simulink model "DC_Simscape_test_no_graphs"  (R2016a)
settings: Solver=ode23t  StartTime=0.0  StopTime=5790*3  MaxStep=0.1  RelTol=1e-3
libraries: nesl_utility x36, fl_lib x33, elec_lib x8, LiBatteryElements_lib x4
settings Model: Creator=Bruno  LastModifiedBy=sara
settings SolverCC: MaxConsecutiveZCs=10000

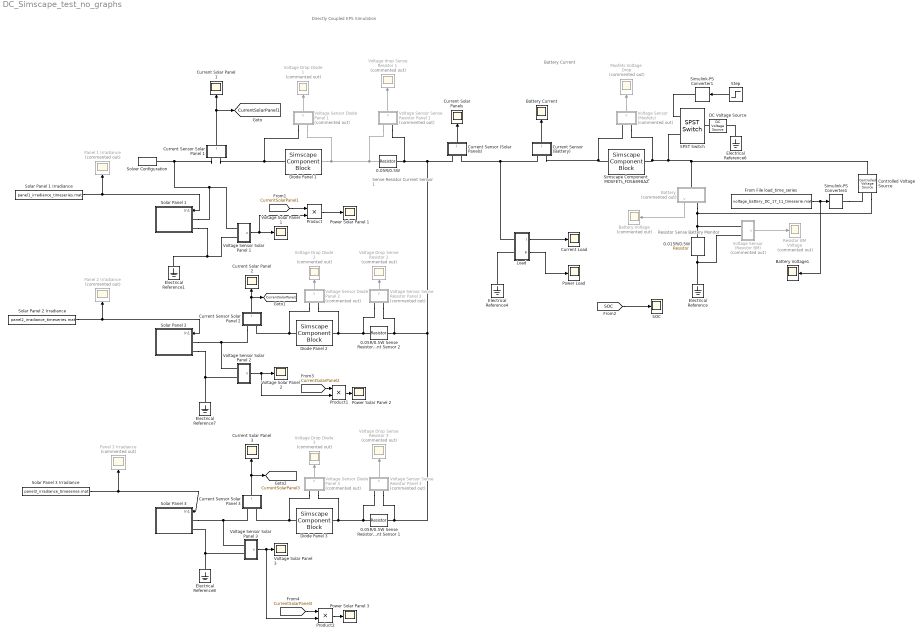
== system DC_Simscape_test_no_graphs ==
  note: Battery Current
  note: Resistor Sense
      | Battery Monitor
  note: Sense Resistor
      | Current Sensor 1
  note: Directly Coupled EPS Simulation
  " Battery" : Subsystem  Commented=on
      settings: CopyFcn=set_param(gcb,'LinkStatus','none')
  " Load" : Subsystem
      settings: CopyFcn=set_param(gcb,'LinkStatus','none')
  " 0.015R/0.5W" : elec_lib/Passive Devices/Resistor  R=0.015 Ohm  R_tol=0.01  enable_R_tol=0  tol_distribution=1  nSigma=4  enable_operating_limits=0  operating_limit_action=2  max_working_voltage=100 V  power_rating=1 W  enable_faults=0  fault_action=1  R_faulted=Inf Ohm  enable_temporal_fault=0  t_fault=1 s  enable_behavioral_fault=0  max_permissible_current=1 A  t_fail_on_current=1 s  noise_mode=0  sample_time=0.001 s  repeatability=1  auto_seed=1471942077  user_seed=0  Tdevice=25 degC  alpha=0.00393 1/K  Tmeas=25 degC  thermal_mass=100 J/K  initial_temperature=25 degC  power_derating_T1=70 degC  power_derating_T2=155 degC  operating_temperature_range_vec=[ -50 150 ] degC
  " 0.05R/0.5W" : elec_lib/Passive Devices/Resistor  R=0.05 Ohm  R_tol=0.01  enable_R_tol=0  tol_distribution=1  nSigma=4  enable_operating_limits=0  operating_limit_action=2  max_working_voltage=100 V  power_rating=1 W  enable_faults=0  fault_action=1  R_faulted=Inf Ohm  enable_temporal_fault=0  t_fault=1 s  enable_behavioral_fault=0  max_permissible_current=1 A  t_fail_on_current=1 s  noise_mode=0  sample_time=0.001 s  repeatability=1  auto_seed=1613585455  user_seed=0  Tdevice=25 degC  alpha=0.00393 1/K  Tmeas=25 degC  thermal_mass=100 J/K  initial_temperature=25 degC  power_derating_T1=70 degC  power_derating_T2=155 degC  operating_temperature_range_vec=[ -50 150 ] degC
  " 0.05R/0.5W Sense Resistor Current Sensor 1" : elec_lib/Passive Devices/Resistor  R=0.05 Ohm  R_tol=0.01  enable_R_tol=0  tol_distribution=1  nSigma=4  enable_operating_limits=0  operating_limit_action=2  max_working_voltage=100 V  power_rating=1 W  enable_faults=0  fault_action=1  R_faulted=Inf Ohm  enable_temporal_fault=0  t_fault=1 s  enable_behavioral_fault=0  max_permissible_current=1 A  t_fail_on_current=1 s  noise_mode=0  sample_time=0.001 s  repeatability=1  auto_seed=4049024516  user_seed=0  Tdevice=25 degC  alpha=0.00393 1/K  Tmeas=25 degC  thermal_mass=100 J/K  initial_temperature=25 degC  power_derating_T1=70 degC  power_derating_T2=155 degC  operating_temperature_range_vec=[ -50 150 ] degC
  " 0.05R/0.5W Sense Resistor Current Sensor 2" : elec_lib/Passive Devices/Resistor  R=0.05 Ohm  R_tol=0.01  enable_R_tol=0  tol_distribution=1  nSigma=4  enable_operating_limits=0  operating_limit_action=2  max_working_voltage=100 V  power_rating=1 W  enable_faults=0  fault_action=1  R_faulted=Inf Ohm  enable_temporal_fault=0  t_fault=1 s  enable_behavioral_fault=0  max_permissible_current=1 A  t_fail_on_current=1 s  noise_mode=0  sample_time=0.001 s  repeatability=1  auto_seed=2353087603  user_seed=0  Tdevice=25 degC  alpha=0.00393 1/K  Tmeas=25 degC  thermal_mass=100 J/K  initial_temperature=25 degC  power_derating_T1=70 degC  power_derating_T2=155 degC  operating_temperature_range_vec=[ -50 150 ] degC
  " Current Solar Panel 1" : Scope
  " Current Solar Panel 2" : Scope
  " Current Solar Panel 3" : Scope
  " Solar Panel 1 Irradiance" : FromFile  FileName=panel1_irradiance_timeseries.mat
  Battery Current : Scope
  Battery Voltage : Scope  Commented=on
  Battery Voltage1 : Scope
  Controlled Voltage Source : fl_lib/Electrical/Electrical Sources/Controlled Voltage Source
  Current Sensor (Battery) : Subsystem
      settings: CopyFcn=set_param(gcb,'LinkStatus','none')
  Current Sensor (Solar Panels) : Subsystem
      settings: CopyFcn=set_param(gcb,'LinkStatus','none')
  Current Sensor Solar Panel 1 : Subsystem
      settings: CopyFcn=set_param(gcb,'LinkStatus','none')
  Current Sensor Solar Panel 2 : Subsystem
      settings: CopyFcn=set_param(gcb,'LinkStatus','none')
  Current Sensor Solar Panel 3 : Subsystem
      settings: CopyFcn=set_param(gcb,'LinkStatus','none')
  Current Solar Panels : Scope
  Current Load : Scope
  DC Voltage Source : fl_lib/Electrical/Electrical Sources/DC Voltage Source  v0=4 V
  Diode Panel 1 : SimscapeComponentBlock  SourceFile=diode_EPS  ComponentPath=diode_EPS  ComponentVariants=diode_EPS  ComponentVariantNames=diode_EPS  ClassName=diode_EPS  SchemaVersion=1  Vt=1.38e-23 * 298 / 1.60e-19 V  R=0.0084 Ohm  n=1.00404  Is=1.3032e-6 A  i_specify=off  i_priority=None  i=1 A  v_specify=off  v_priority=None  v=0 V
      settings: CopyFcn=simscape.engine.sli.internal.componentblockcallback(gcbh,'COPY')  PreCopyFcn=simscape.engine.sli.internal.componentblockcallback(gcbh,'PRECOPY')  PreDeleteFcn=simscape.engine.sli.internal.componentblockcallback(gcbh,'PREDELETE')
      mask Type: Code produced by Embedded Systems Group - UFSC
      mask Display:
      | disp('Simscape\n\n\n')
      | disp('\n\n\ndiode_EPS');
      | color('red');
      | port_label('RConn', 1,'-');
      | port_label('LConn', 1,'+');
  Diode Panel 2 : SimscapeComponentBlock  SourceFile=diode_EPS  ComponentPath=diode_EPS  ComponentVariants=diode_EPS  ComponentVariantNames=diode_EPS  ClassName=diode_EPS  SchemaVersion=1  Vt=1.38e-23 * 298 / 1.60e-19 V  R=0.0084 Ohm  n=1.00404  Is=1.3032e-6 A  i_specify=off  i_priority=None  i=1 A  v_specify=off  v_priority=None  v=0 V
      settings: CopyFcn=simscape.engine.sli.internal.componentblockcallback(gcbh,'COPY')  PreCopyFcn=simscape.engine.sli.internal.componentblockcallback(gcbh,'PRECOPY')  PreDeleteFcn=simscape.engine.sli.internal.componentblockcallback(gcbh,'PREDELETE')
      mask Type: Code produced by Embedded Systems Group - UFSC
      mask Display:
      | disp('Simscape\n\n\n')
      | disp('\n\n\ndiode_EPS');
      | color('red');
      | port_label('RConn', 1,'-');
      | port_label('LConn', 1,'+');
  Diode Panel 3 : SimscapeComponentBlock  SourceFile=diode_EPS  ComponentPath=diode_EPS  ComponentVariants=diode_EPS  ComponentVariantNames=diode_EPS  ClassName=diode_EPS  SchemaVersion=1  Vt=1.38e-23 * 298 / 1.60e-19 V  R=0.0084 Ohm  n=1.00404  Is=1.3032e-6 A  i_specify=off  i_priority=None  i=1 A  v_specify=off  v_priority=None  v=0 V
      settings: CopyFcn=simscape.engine.sli.internal.componentblockcallback(gcbh,'COPY')  PreCopyFcn=simscape.engine.sli.internal.componentblockcallback(gcbh,'PRECOPY')  PreDeleteFcn=simscape.engine.sli.internal.componentblockcallback(gcbh,'PREDELETE')
      mask Type: Code produced by Embedded Systems Group - UFSC
      mask Display:
      | disp('Simscape\n\n\n')
      | disp('\n\n\ndiode_EPS');
      | color('red');
      | port_label('RConn', 1,'-');
      | port_label('LConn', 1,'+');
  Electrical Reference{,1,4,6..8} (6 alike) : fl_lib/Electrical/Electrical Elements/Electrical Reference
  From File load_time_series : FromFile  FileName=voltage_battery_DC_17_11_timeserie.mat  SampleTime=1
  Mosfets Voltage Drop : Scope  Commented=on
  Panel 1 Irradiance : Scope  Commented=on
  Panel 2 Irradiance : Scope  Commented=on
  Panel 3 Irradiance : Scope  Commented=on
  Power Solar Panel 1 : Scope
  Power Solar Panel 2 : Scope
  Power Solar Panel 3 : Scope
  Power Load : Scope
  Product : Product
  Product1 : Product
  Product2 : Product
  Resistor BM Voltage : Scope  Commented=on
  SOC : Scope
  SPST Switch : elec_lib/Passive Devices/Switches/SPST Switch  R_closed=0.01 Ohm  G_open=1e-6 S  Threshold=0 V  Width=0 V  model_dynamics=0  t_on=0.001 s  t_off=0.001 s  initial_vT=0 V
  Simscape Component_MOSFETs_FDS6898AZ : SimscapeComponentBlock  SourceFile=MOSFETs_EPS  ComponentPath=MOSFETs_EPS  ComponentVariants=MOSFETs_EPS  ComponentVariantNames=MOSFETs_EPS  ClassName=MOSFETs_EPS  SchemaVersion=1  Vt=1.38e-23 * 298 / 1.60e-19 V  Rsd=0.27 Ohm  Rs=0.008235 Ohm  n=1.89492  Is=1.26064e-7 A  i_specify=on  i_priority=None  i=1 A  v_specify=on  v_priority=None  v=4 V  Vr_DC_specify=on  Vr_DC_priority=None  Vr_DC=1 V  Vr_CC_specify=on  Vr_CC_priority=None  Vr_CC=1 V
      settings: CopyFcn=simscape.engine.sli.internal.componentblockcallback(gcbh,'COPY')  PreCopyFcn=simscape.engine.sli.internal.componentblockcallback(gcbh,'PRECOPY')  PreDeleteFcn=simscape.engine.sli.internal.componentblockcallback(gcbh,'PREDELETE')
      mask Type: Code produced by Embedded Systems Group - UFSC
      mask Display:
      | disp('Simscape\n\n\n')
      | disp('\n\n\nMOSFETs_EPS');
      | color('red');
      | port_label('RConn', 1,'-');
      | port_label('LConn', 1,'+');
  Simulink-PS Converter1 : nesl_utility/Simulink-PS Converter  PhysicalDomain=network_engine_domain  SubClassName=ps_input  LeftPortType=input  RightPortType=output  PseudoPeriodic=off  Frequencies=[]  NoiseDistribution=none  NoiseParameters=[]  Unit=1  AffineConversion=off  InputFiltering=off  SimscapeFilterOrder=1  InputFilterTimeConstant=0.001  UdotUserProvided=1
  Simulink-PS Converter4 : nesl_utility/Simulink-PS Converter  PhysicalDomain=network_engine_domain  SubClassName=ps_input  LeftPortType=input  RightPortType=output  PseudoPeriodic=off  Frequencies=[]  NoiseDistribution=none  NoiseParameters=[]  Unit=1  AffineConversion=off  InputFiltering=off  SimscapeFilterOrder=1  InputFilterTimeConstant=0.001  UdotUserProvided=1
  Solar Panel 1 : Subsystem
      settings: CopyFcn=set_param(gcb,'LinkStatus','none')
  Solar Panel 2 : Subsystem
      settings: CopyFcn=set_param(gcb,'LinkStatus','none')
  Solar Panel 2 Irradiance : FromFile  FileName=panel2_irradiance_timeseries.mat
  Solar Panel 3 : Subsystem
      settings: CopyFcn=set_param(gcb,'LinkStatus','none')
  Solar Panel 3 Irradiance : FromFile  FileName=panel3_irradiance_timeseries.mat
  Solver Configuration : nesl_utility/Solver Configuration  PhysicalDomain=network_engine_domain  SubClassName=solver  LeftPortType=input  RightPortType=generic  Accelerate=off  Tones=[]  Harmonics=[]  SimulateNoise=off  Profile=off  UseLocalSampling=off  EnableSwitchedLinearOptims=on  FrequencyDomain=off  UseCCode=off  RelTol=0.001  AbsTol=1e-06  MinStep=1e-09  ToWorkspace=off  RevertToSquareIcSolve=off  NumHomotopyIterations=100  PhasorMode=off  PhasorModeNumHarmonics=1  OverrideAbsTol=off  DoDC=off  ResidualTolerance=1e-3  UseLocalSolver=off  LocalSolverChoice=NE_BACKWARD_EULER_ADVANCER  LocalSolverSampleTime=.001  DoFixedCost=off  MaxNonlinIter=3  MaxModeIter=2  LinearAlgebra=Sparse  DelaysMemoryBudget=1024  AutomaticFiltering=on  FilteringTimeConstant=0.001
  Step : Step  Before=1  After=0  SampleTime=0
  Voltage Sensor (Mosfets) : Subsystem  Commented=on
      settings: CopyFcn=set_param(gcb,'LinkStatus','none')
  Voltage Sensor (Resistor BM) : Subsystem  Commented=on
      settings: CopyFcn=set_param(gcb,'LinkStatus','none')
  Voltage Solar Panel 1 : Scope
  Voltage Solar Panel 2 : Scope
  Voltage Solar Panel 3 : Scope
  "Voltage Drop Diode 1 " : Scope  Commented=on
  Voltage Drop Diode 2 : Scope  Commented=on
  Voltage Drop Diode 3 : Scope  Commented=on
  Voltage Drop Sense Resistor 2 : Scope  Commented=on
  Voltage Drop Sense Resistor 3 : Scope  Commented=on
  Voltage Sensor Diode Panel 1 : Subsystem  Commented=on
      settings: CopyFcn=set_param(gcb,'LinkStatus','none')
  Voltage Sensor Diode Panel 2 : Subsystem  Commented=on
      settings: CopyFcn=set_param(gcb,'LinkStatus','none')
  Voltage Sensor Diode Panel 3 : Subsystem  Commented=on
      settings: CopyFcn=set_param(gcb,'LinkStatus','none')
  "Voltage Sensor Sense Resistor Panel 1 " : Subsystem  Commented=on
      settings: CopyFcn=set_param(gcb,'LinkStatus','none')
  Voltage Sensor Sense Resistor Panel 2 : Subsystem  Commented=on
      settings: CopyFcn=set_param(gcb,'LinkStatus','none')
  Voltage Sensor Sense Resistor Panel 3 : Subsystem  Commented=on
      settings: CopyFcn=set_param(gcb,'LinkStatus','none')
  Voltage Sensor Solar Panel 1 : Subsystem
      settings: CopyFcn=set_param(gcb,'LinkStatus','none')
  Voltage Sensor Solar Panel 2 : Subsystem
      settings: CopyFcn=set_param(gcb,'LinkStatus','none')
  Voltage Sensor Solar Panel 3 : Subsystem
      settings: CopyFcn=set_param(gcb,'LinkStatus','none')
  Voltage drop Sense Resistor 1 : Scope  Commented=on
  tag scope: CurrentSolarPanel1=global, CurrentSolarPanel2=global, CurrentSolarPanel3=global
  wires:
  Voltage Sensor (Mosfets)/1(v) -> Mosfets Voltage Drop/1
  Voltage Sensor Diode Panel 1/1(v) -> "Voltage Drop Diode 1 "/1
  Current Sensor (Solar Panels)/1(i) -> Current Solar Panels/1
  "Voltage Sensor Sense Resistor Panel 1 "/1(v) -> Voltage drop Sense Resistor 1/1
  Voltage Sensor (Resistor BM)/1(v) -> Resistor BM Voltage/1
  Voltage Sensor Solar Panel 1/1(v) -> Product/2, Voltage Solar Panel 1/1
  Current Sensor (Battery)/1(i) -> Battery Current/1
  Current Sensor Solar Panel 1/1(i) -> [CurrentSolarPanel1], " Current Solar Panel 1"/1
  Step/1 -> Simulink-PS Converter1/1
  Product/1 -> Power Solar Panel 1/1
  " Solar Panel 1 Irradiance"/1 -> Solar Panel 1/1(In1), Panel 1 Irradiance/1
  Solar Panel 2 Irradiance/1 -> Panel 2 Irradiance/1, Solar Panel 2/1(In1)
  Voltage Sensor Solar Panel 2/1(v) -> Product1/2, Voltage Solar Panel 2/1
  Voltage Sensor Diode Panel 2/1(v) -> Voltage Drop Diode 2/1
  Voltage Sensor Sense Resistor Panel 2/1(v) -> Voltage Drop Sense Resistor 2/1
  Solar Panel 3 Irradiance/1 -> Panel 3 Irradiance/1, Solar Panel 3/1(In1)
  Voltage Sensor Diode Panel 3/1(v) -> Voltage Drop Diode 3/1
  Current Sensor Solar Panel 3/1(i) -> [CurrentSolarPanel3], " Current Solar Panel 3"/1
  " Load"/1(I) -> Current Load/1
  " Load"/2(P) -> Power Load/1
  " Battery"/1(v) -> Battery Voltage/1
  [SOC] -> SOC/1
  Voltage Sensor Sense Resistor Panel 3/1(v) -> Voltage Drop Sense Resistor 3/1
  Current Sensor Solar Panel 2/1(i) -> [CurrentSolarPanel2], " Current Solar Panel 2"/1
  [CurrentSolarPanel1] -> Product/1
  Product1/1 -> Power Solar Panel 2/1
  [CurrentSolarPanel2] -> Product1/1
  Voltage Sensor Solar Panel 3/1(v) -> Product2/2, Voltage Solar Panel 3/1
  Product2/1 -> Power Solar Panel 3/1
  [CurrentSolarPanel3] -> Product2/1
  From File load_time_series/1 -> Battery Voltage1/1, Simulink-PS Converter4/1
  connections:
  Current Sensor Solar Panel 1/LConn2 -- Voltage Sensor Diode Panel 1/LConn1 -- Diode Panel 1/LConn1
  " 0.015R/0.5W"/LConn1 -- Controlled Voltage Source/RConn2 -- " Battery"/RConn1 -- Voltage Sensor (Resistor BM)/LConn1
  Voltage Sensor Diode Panel 1/LConn2 -- Diode Panel 1/RConn1 -- "Voltage Sensor Sense Resistor Panel 1 "/LConn1 -- " 0.05R/0.5W"/LConn1
  Voltage Sensor (Mosfets)/LConn1 -- Simscape Component_MOSFETs_FDS6898AZ/LConn1 -- Current Sensor (Battery)/LConn2
  " 0.05R/0.5W"/RConn1 -- Voltage Sensor Sense Resistor Panel 3/LConn2 -- " 0.05R/0.5W Sense Resistor Current Sensor 1"/RConn1 -- Voltage Sensor Sense Resistor Panel 2/LConn2 -- " 0.05R/0.5W Sense Resistor Current Sensor 2"/RConn1 -- Current Sensor (Solar Panels)/LConn1 -- "Voltage Sensor Sense Resistor Panel 1 "/LConn2
  Solver Configuration/RConn1 -- Solar Panel 1/LConn1 -- Voltage Sensor Solar Panel 1/LConn1 -- Current Sensor Solar Panel 1/LConn1
  Current Sensor (Battery)/LConn1 -- " Load"/LConn1 -- Current Sensor (Solar Panels)/LConn2
  " 0.015R/0.5W"/RConn1 -- Voltage Sensor (Resistor BM)/LConn2 -- Electrical Reference/LConn1
  Simscape Component_MOSFETs_FDS6898AZ/RConn1 -- Controlled Voltage Source/LConn1 -- " Battery"/LConn1 -- SPST Switch/LConn2 -- Voltage Sensor (Mosfets)/LConn2
  Voltage Sensor Solar Panel 1/LConn2 -- Electrical Reference1/LConn1 -- Solar Panel 1/LConn2
  Simulink-PS Converter1/RConn1 -- SPST Switch/LConn1
  Electrical Reference6/LConn1 -- DC Voltage Source/RConn1
  DC Voltage Source/LConn1 -- SPST Switch/RConn1
  Solar Panel 2/LConn2 -- Electrical Reference7/LConn1 -- Voltage Sensor Solar Panel 2/LConn2
  Solar Panel 2/LConn1 -- Current Sensor Solar Panel 2/LConn1 -- Voltage Sensor Solar Panel 2/LConn1
  " 0.05R/0.5W Sense Resistor Current Sensor 2"/LConn1 -- Voltage Sensor Sense Resistor Panel 2/LConn1 -- Voltage Sensor Diode Panel 2/LConn2 -- Diode Panel 2/RConn1
  Diode Panel 2/LConn1 -- Voltage Sensor Diode Panel 2/LConn1 -- Current Sensor Solar Panel 2/LConn2
  Solar Panel 3/LConn1 -- Voltage Sensor Solar Panel 3/LConn1 -- Current Sensor Solar Panel 3/LConn1
  Electrical Reference8/LConn1 -- Voltage Sensor Solar Panel 3/LConn2 -- Solar Panel 3/LConn2
  Diode Panel 3/LConn1 -- Current Sensor Solar Panel 3/LConn2 -- Voltage Sensor Diode Panel 3/LConn1
  " 0.05R/0.5W Sense Resistor Current Sensor 1"/LConn1 -- Voltage Sensor Sense Resistor Panel 3/LConn1 -- Voltage Sensor Diode Panel 3/LConn2 -- Diode Panel 3/RConn1
  " Load"/LConn2 -- Electrical Reference4/LConn1
  Simulink-PS Converter4/RConn1 -- Controlled Voltage Source/RConn1

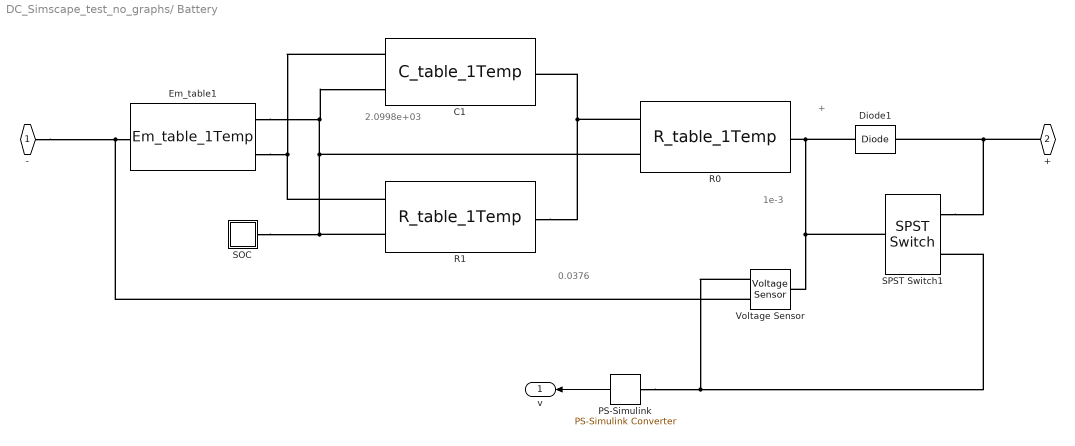
== system DC_Simscape_test_no_graphs/ Battery ==
  note: 1e-3
  note: 0.0376
  note: 2.0998e+03
  note: +
  " SOC " : Subsystem
  C1 : LiBatteryElements_lib/C_table_1Temp  C_Table=2.0998e+03*ones(5, 1) F  SOC_Table=[0.0; 0.1; 0.5; 0.9; 1.0]  v0=0 V
  Diode1 : fl_lib/Electrical/Electrical Elements/Diode  Vf=0.0001 V  Ron=0.0001 Ohm  Goff=1e-8 1/Ohm  i_specify=off  i_priority=None  i=0 A  v_specify=off  v_priority=None  v=0 V
  Em_table1 : LiBatteryElements_lib/Em_table_1Temp  Em_Table=[2.387048;3.045524;3.235201;3.386789;3.465654;3.531649;3.574124;3.602364;3.63132;3.666658;3.730669;3.801663;3.889973;3.927882;4.143995] V  SOC_Table=[0;0.010;0.025;0.050;0.100;0.200;0.300;0.400;0.500;0.600;0.700;0.800;0.900;0.950;1.000]  C=2.4566 hr*A  Qinit=0 hr*A
  PS-Simulink : nesl_utility/PS-Simulink Converter  PhysicalDomain=network_engine_domain  SubClassName=ps_output  LeftPortType=input  RightPortType=output  PseudoPeriodic=off  Frequencies=[]  Unit=V  AffineConversion=off
  R0 : LiBatteryElements_lib/R_table_1Temp  R_Table=1e-3*ones(5, 1) Ohm  SOC_Table=[0.0; 0.1; 0.5; 0.9; 1.0]
  R1 : LiBatteryElements_lib/R_table_1Temp  R_Table=0.0376*ones(5, 1) Ohm  SOC_Table=[0.0; 0.1; 0.5; 0.9; 1.0]
  SPST Switch1 : elec_lib/Passive Devices/Switches/SPST Switch  R_closed=0.001 Ohm  G_open=1e-6 S  Threshold=2.4 V  Width=0.1 V  model_dynamics=0  t_on=0.001 s  t_off=0.001 s  initial_vT=0 V
  Voltage Sensor : fl_lib/Electrical/Electrical Sensors/Voltage Sensor
  - : PMIOPort  Port=1  Side=Right
  + : PMIOPort  Port=2  Side=Left
  v : Outport
  wires:
  PS-Simulink/1 -> v/1
  connections:
  SPST Switch1/LConn2 -- Diode1/LConn1 -- +/RConn1
  R1/LConn2 -- " SOC "/LConn1 -- R0/LConn2 -- Em_table1/LConn2 -- C1/LConn2
  Voltage Sensor/RConn1 -- SPST Switch1/LConn1 -- PS-Simulink/LConn1
  R0/RConn1 -- SPST Switch1/RConn1 -- Voltage Sensor/LConn1 -- Diode1/RConn1
  Voltage Sensor/RConn2 -- Em_table1/RConn1 -- -/RConn1
  R1/RConn1 -- R0/LConn1 -- C1/RConn1
  R1/LConn1 -- Em_table1/LConn1 -- C1/LConn1

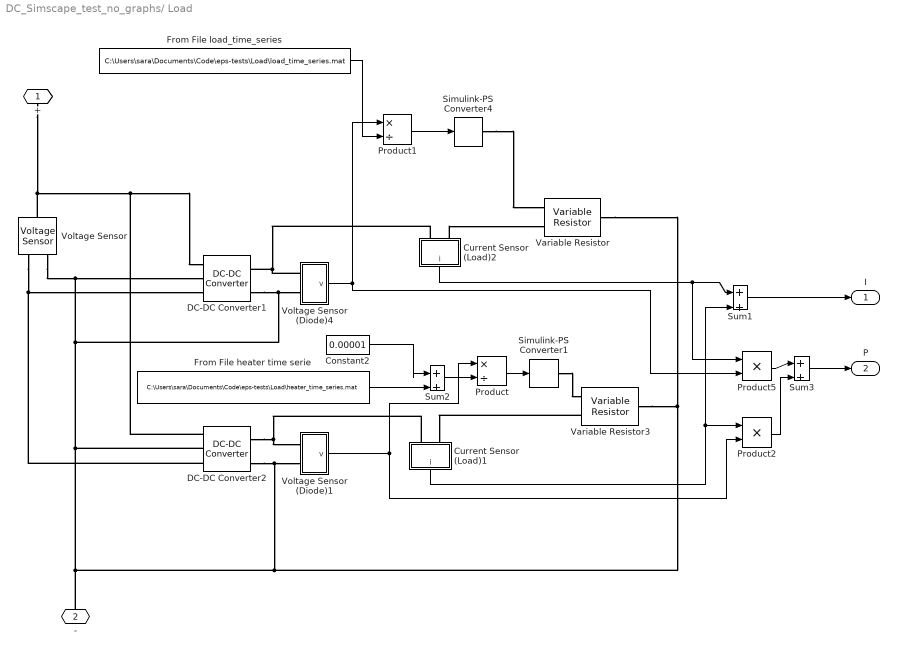
== system DC_Simscape_test_no_graphs/ Load ==
  Constant2 : Constant  Value=0.00001
  Current Sensor (Load)1 : Subsystem
      settings: CopyFcn=set_param(gcb,'LinkStatus','none')
  Current Sensor (Load)2 : Subsystem
      settings: CopyFcn=set_param(gcb,'LinkStatus','none')
  DC-DC Converter1 : elec_lib/Sources/DC-DC Converter  v_ref=5 V  P_rated=10 W  droop_param=1  droop=0.0 V/A  droop_percent=2  reversible=0  efficiency=99.9999  P_fixed=0.0001 mW  model_dynamics=0  tau=1 s  v_ini=5 V  i1_max=10 A  fault_condition=2  fault_threshold=2.5  R_fixed=100 Ohm  R_out=0.1 Ohm  fault_sign=1
  DC-DC Converter2 : elec_lib/Sources/DC-DC Converter  v_ref=5 V  P_rated=10 W  droop_param=1  droop=0.0 V/A  droop_percent=2  reversible=0  efficiency=99.9999  P_fixed=0.0001 mW  model_dynamics=0  tau=1 s  v_ini=5 V  i1_max=10 A  fault_condition=2  fault_threshold=2.5  R_fixed=100 Ohm  R_out=0.1 Ohm  fault_sign=1
  From File heater time serie : FromFile  FileName=C:\Users\sara\Documents\Code\eps-tests\Load\heater_time_series.mat
  From File load_time_series : FromFile  FileName=C:\Users\sara\Documents\Code\eps-tests\Load\load_time_series.mat
  Product : Product  Inputs=*/  InputSameDT=on
  Product1 : Product  Inputs=*/  InputSameDT=on
  Product2 : Product
  Product5 : Product
  Simulink-PS Converter1 : nesl_utility/Simulink-PS Converter  PhysicalDomain=network_engine_domain  SubClassName=ps_input  LeftPortType=input  RightPortType=output  PseudoPeriodic=off  Frequencies=[]  NoiseDistribution=none  NoiseParameters=[]  Unit=1  AffineConversion=off  InputFiltering=off  SimscapeFilterOrder=1  InputFilterTimeConstant=0.001  UdotUserProvided=1
  Simulink-PS Converter4 : nesl_utility/Simulink-PS Converter  PhysicalDomain=network_engine_domain  SubClassName=ps_input  LeftPortType=input  RightPortType=output  PseudoPeriodic=off  Frequencies=[]  NoiseDistribution=none  NoiseParameters=[]  Unit=1  AffineConversion=off  InputFiltering=off  SimscapeFilterOrder=1  InputFilterTimeConstant=0.001  UdotUserProvided=1
  Sum1 : Sum  Inputs=|++
  Sum2 : Sum  Inputs=|++
  Sum3 : Sum  Inputs=|++
  Variable Resistor : fl_lib/Electrical/Electrical Elements/Variable Resistor  Rmin=9.598742 Ohm  i_specify=off  i_priority=None  i=0 A  v_specify=off  v_priority=None  v=0 V
  Variable Resistor3 : fl_lib/Electrical/Electrical Elements/Variable Resistor  Rmin=7.861635 Ohm  i_specify=off  i_priority=None  i=0 A  v_specify=off  v_priority=None  v=0 V
  Voltage Sensor (Diode)1 : Subsystem
      settings: CopyFcn=set_param(gcb,'LinkStatus','none')
  Voltage Sensor (Diode)4 : Subsystem
      settings: CopyFcn=set_param(gcb,'LinkStatus','none')
  Voltage Sensor : fl_lib/Electrical/Electrical Sensors/Voltage Sensor
  + : PMIOPort  Port=1  Side=Left
  - : PMIOPort  Port=2  Side=Left
  I : Outport
  P : Outport  Port=2
  wires:
  From File load_time_series/1 -> Product1/2
  Voltage Sensor (Diode)4/1(v) -> Product1/1, Product5/2
  Product1/1 -> Simulink-PS Converter4/1
  Voltage Sensor (Diode)1/1(v) -> Product/1, Product2/2
  Constant2/1 -> Sum2/1
  Current Sensor (Load)2/1(i) -> Product5/1, Sum1/1
  Current Sensor (Load)1/1(i) -> Product2/1, Sum1/2
  Sum1/1 -> I/1
  Product5/1 -> Sum3/1
  Product2/1 -> Sum3/2
  Sum3/1 -> P/1
  From File heater time serie/1 -> Sum2/2
  Sum2/1 -> Product/2
  Product/1 -> Simulink-PS Converter1/1
  connections:
  Voltage Sensor (Diode)4/LConn1 -- DC-DC Converter1/RConn1 -- Current Sensor (Load)2/LConn1
  Current Sensor (Load)2/LConn2 -- Variable Resistor/LConn2
  Simulink-PS Converter4/RConn1 -- Variable Resistor/LConn1
  +/RConn1 -- Voltage Sensor/LConn1 -- DC-DC Converter2/LConn1 -- DC-DC Converter1/LConn1
  DC-DC Converter2/RConn2 -- Voltage Sensor (Diode)4/LConn2 -- DC-DC Converter1/RConn2 -- DC-DC Converter1/LConn2 -- Voltage Sensor/RConn2 -- DC-DC Converter2/LConn2 -- -/RConn1 -- Variable Resistor/RConn1 -- Variable Resistor3/RConn1 -- Voltage Sensor (Diode)1/LConn2
  Voltage Sensor/RConn1 -- DC-DC Converter2/LConn3 -- DC-DC Converter1/LConn3
  DC-DC Converter2/RConn1 -- Voltage Sensor (Diode)1/LConn1 -- Current Sensor (Load)1/LConn1
  Variable Resistor3/LConn2 -- Current Sensor (Load)1/LConn2
  Simulink-PS Converter1/RConn1 -- Variable Resistor3/LConn1

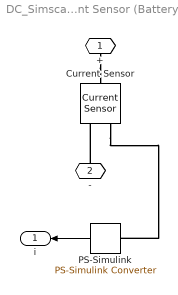
== system DC_Simscape_test_no_graphs/Current Sensor (Battery) ==
  Current Sensor : fl_lib/Electrical/Electrical Sensors/Current Sensor
  PS-Simulink : nesl_utility/PS-Simulink Converter  PhysicalDomain=network_engine_domain  SubClassName=ps_output  LeftPortType=input  RightPortType=output  PseudoPeriodic=off  Frequencies=[]  Unit=A  AffineConversion=off
  + : PMIOPort  Port=1  Side=Left
  - : PMIOPort  Port=2  Side=Left
  i : Outport
  wires:
  PS-Simulink/1 -> i/1
  connections:
  -/RConn1 -- Current Sensor/RConn2
  +/RConn1 -- Current Sensor/LConn1
  Current Sensor/RConn1 -- PS-Simulink/LConn1

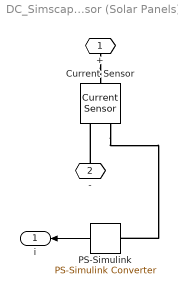
== system DC_Simscape_test_no_graphs/Current Sensor (Solar Panels) ==
  Current Sensor : fl_lib/Electrical/Electrical Sensors/Current Sensor
  PS-Simulink : nesl_utility/PS-Simulink Converter  PhysicalDomain=network_engine_domain  SubClassName=ps_output  LeftPortType=input  RightPortType=output  PseudoPeriodic=off  Frequencies=[]  Unit=A  AffineConversion=off
  + : PMIOPort  Port=1  Side=Left
  - : PMIOPort  Port=2  Side=Left
  i : Outport
  wires:
  PS-Simulink/1 -> i/1
  connections:
  -/RConn1 -- Current Sensor/RConn2
  +/RConn1 -- Current Sensor/LConn1
  Current Sensor/RConn1 -- PS-Simulink/LConn1

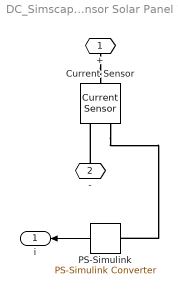
== system DC_Simscape_test_no_graphs/Current Sensor Solar Panel 1 ==
  Current Sensor : fl_lib/Electrical/Electrical Sensors/Current Sensor
  PS-Simulink : nesl_utility/PS-Simulink Converter  PhysicalDomain=network_engine_domain  SubClassName=ps_output  LeftPortType=input  RightPortType=output  PseudoPeriodic=off  Frequencies=[]  Unit=A  AffineConversion=off
  + : PMIOPort  Port=1  Side=Left
  - : PMIOPort  Port=2  Side=Left
  i : Outport
  wires:
  PS-Simulink/1 -> i/1
  connections:
  -/RConn1 -- Current Sensor/RConn2
  +/RConn1 -- Current Sensor/LConn1
  Current Sensor/RConn1 -- PS-Simulink/LConn1

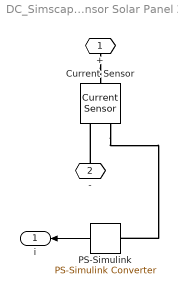
== system DC_Simscape_test_no_graphs/Current Sensor Solar Panel 2 ==
  Current Sensor : fl_lib/Electrical/Electrical Sensors/Current Sensor
  PS-Simulink : nesl_utility/PS-Simulink Converter  PhysicalDomain=network_engine_domain  SubClassName=ps_output  LeftPortType=input  RightPortType=output  PseudoPeriodic=off  Frequencies=[]  Unit=A  AffineConversion=off
  + : PMIOPort  Port=1  Side=Left
  - : PMIOPort  Port=2  Side=Left
  i : Outport
  wires:
  PS-Simulink/1 -> i/1
  connections:
  -/RConn1 -- Current Sensor/RConn2
  +/RConn1 -- Current Sensor/LConn1
  Current Sensor/RConn1 -- PS-Simulink/LConn1

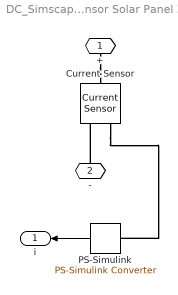
== system DC_Simscape_test_no_graphs/Current Sensor Solar Panel 3 ==
  Current Sensor : fl_lib/Electrical/Electrical Sensors/Current Sensor
  PS-Simulink : nesl_utility/PS-Simulink Converter  PhysicalDomain=network_engine_domain  SubClassName=ps_output  LeftPortType=input  RightPortType=output  PseudoPeriodic=off  Frequencies=[]  Unit=A  AffineConversion=off
  + : PMIOPort  Port=1  Side=Left
  - : PMIOPort  Port=2  Side=Left
  i : Outport
  wires:
  PS-Simulink/1 -> i/1
  connections:
  -/RConn1 -- Current Sensor/RConn2
  +/RConn1 -- Current Sensor/LConn1
  Current Sensor/RConn1 -- PS-Simulink/LConn1

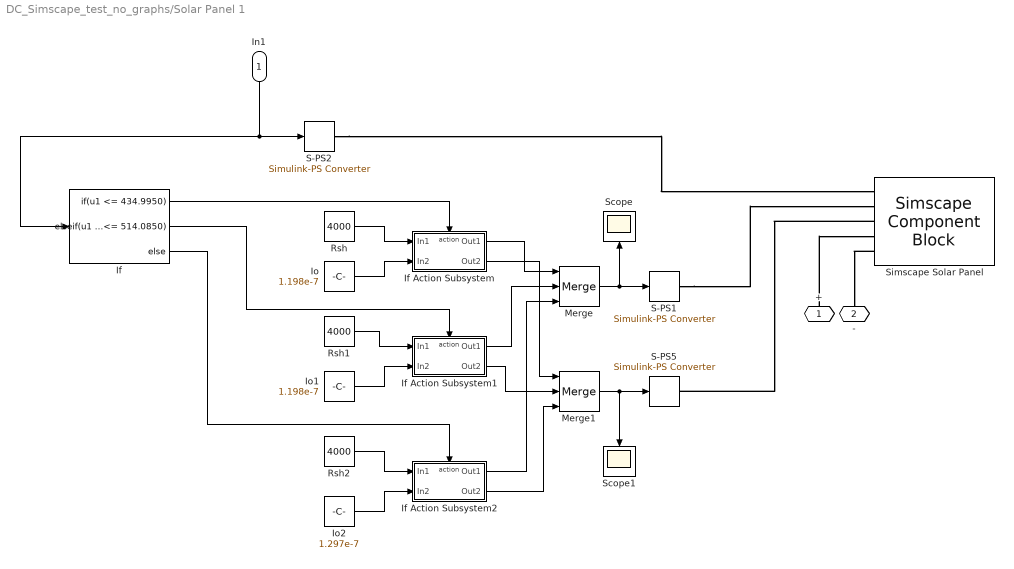
== system DC_Simscape_test_no_graphs/Solar Panel 1 ==
  In1 : Inport
  If : If  IfExpression=u1 <= 434.9950  ElseIfExpressions=u1 <= 514.0850
  If Action Subsystem : Subsystem  TreatAsAtomicUnit=on
  If Action Subsystem1 : Subsystem  TreatAsAtomicUnit=on
  If Action Subsystem2 : Subsystem  TreatAsAtomicUnit=on
  Io : Constant  Value=1.198e-7
  Io1 : Constant  Value=1.198e-7
  Io2 : Constant  Value=1.297e-7
  Merge : Merge  Inputs=3
  Merge1 : Merge  Inputs=3
  Rsh : Constant  Value=4000
  Rsh1 : Constant  Value=4000
  Rsh2 : Constant  Value=4000
  S-PS1 : nesl_utility/Simulink-PS Converter  PhysicalDomain=network_engine_domain  SubClassName=ps_input  LeftPortType=input  RightPortType=output  PseudoPeriodic=off  Frequencies=[]  NoiseDistribution=none  NoiseParameters=[]  Unit=1  AffineConversion=off  InputFiltering=off  SimscapeFilterOrder=1  InputFilterTimeConstant=0.001  UdotUserProvided=1
  S-PS2 : nesl_utility/Simulink-PS Converter  PhysicalDomain=network_engine_domain  SubClassName=ps_input  LeftPortType=input  RightPortType=output  PseudoPeriodic=off  Frequencies=[]  NoiseDistribution=none  NoiseParameters=[]  Unit=1  AffineConversion=off  InputFiltering=off  SimscapeFilterOrder=1  InputFilterTimeConstant=0.001  UdotUserProvided=1
  S-PS5 : nesl_utility/Simulink-PS Converter  PhysicalDomain=network_engine_domain  SubClassName=ps_input  LeftPortType=input  RightPortType=output  PseudoPeriodic=off  Frequencies=[]  NoiseDistribution=none  NoiseParameters=[]  Unit=1  AffineConversion=off  InputFiltering=off  SimscapeFilterOrder=1  InputFilterTimeConstant=0.001  UdotUserProvided=1
  Scope : Scope
  Scope1 : Scope
  Simscape Solar Panel : SimscapeComponentBlock  SourceFile=simscape.solarPanel  ComponentPath=simscape.solarPanel  ComponentVariants=simscape.solarPanel  ComponentVariantNames=solarPanel  ClassName=solarPanel  SchemaVersion=1  Rs=1 Ohm  A=2  Iph0=0.050 A  Np=5  Ns=8  Npp=1  efficiency=0.93  i_specify=off  i_priority=None  i=0 A  v_specify=off  v_priority=None  v=0 V
      settings: CopyFcn=simscape.engine.sli.internal.componentblockcallback(gcbh,'COPY')  PreCopyFcn=simscape.engine.sli.internal.componentblockcallback(gcbh,'PRECOPY')  PreDeleteFcn=simscape.engine.sli.internal.componentblockcallback(gcbh,'PREDELETE')
      mask Type: solarPanel
      mask Display:
      | disp('Simscape\n\n\n')
      | disp('\n\n\nsolarPanel');
      | color('red');
      | port_label('LConn', 5,'n');
      | port_label('LConn', 4,'p');
      | port_label('LConn', 3,'diode saturation current');
      | port_label('LConn', 2,'parallel resistance');
      | port_label('LConn', 1,'I');
  + : PMIOPort  Port=1  Side=Left
  - : PMIOPort  Port=2  Side=Left
  wires:
  In1/1 -> If/1, S-PS2/1
  If/1 -> If Action Subsystem/Action
  Rsh/1 -> If Action Subsystem/1(In1)
  Io/1 -> If Action Subsystem/2(In2)
  If/2 -> If Action Subsystem1/Action
  Io1/1 -> If Action Subsystem1/2(In2)
  Rsh1/1 -> If Action Subsystem1/1(In1)
  If Action Subsystem1/1(Out1) -> Merge/2
  If Action Subsystem/1(Out1) -> Merge/1
  Merge/1 -> Scope/1, S-PS1/1
  If/3 -> If Action Subsystem2/Action
  Rsh2/1 -> If Action Subsystem2/1(In1)
  Io2/1 -> If Action Subsystem2/2(In2)
  If Action Subsystem2/1(Out1) -> Merge/3
  If Action Subsystem/2(Out2) -> Merge1/1
  If Action Subsystem1/2(Out2) -> Merge1/2
  If Action Subsystem2/2(Out2) -> Merge1/3
  Merge1/1 -> Scope1/1, S-PS5/1
  connections:
  +/RConn1 -- Simscape Solar Panel/LConn4
  Simscape Solar Panel/LConn5 -- -/RConn1
  S-PS1/RConn1 -- Simscape Solar Panel/LConn2
  Simscape Solar Panel/LConn3 -- S-PS5/RConn1
  S-PS2/RConn1 -- Simscape Solar Panel/LConn1

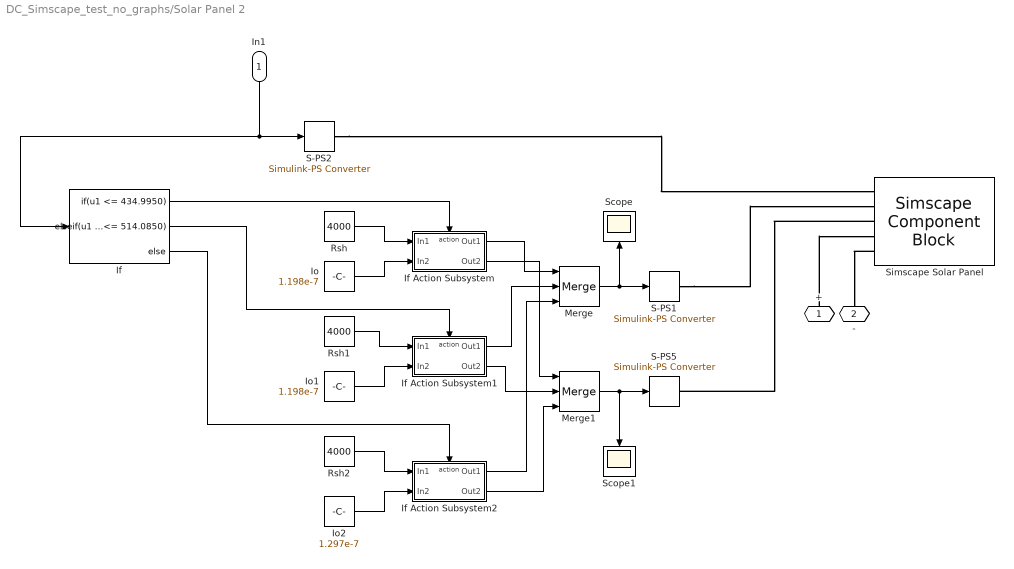
== system DC_Simscape_test_no_graphs/Solar Panel 2 ==
  In1 : Inport
  If : If  IfExpression=u1 <= 434.9950  ElseIfExpressions=u1 <= 514.0850
  If Action Subsystem : Subsystem  TreatAsAtomicUnit=on
  If Action Subsystem1 : Subsystem  TreatAsAtomicUnit=on
  If Action Subsystem2 : Subsystem  TreatAsAtomicUnit=on
  Io : Constant  Value=1.198e-7
  Io1 : Constant  Value=1.198e-7
  Io2 : Constant  Value=1.297e-7
  Merge : Merge  Inputs=3
  Merge1 : Merge  Inputs=3
  Rsh : Constant  Value=4000
  Rsh1 : Constant  Value=4000
  Rsh2 : Constant  Value=4000
  S-PS1 : nesl_utility/Simulink-PS Converter  PhysicalDomain=network_engine_domain  SubClassName=ps_input  LeftPortType=input  RightPortType=output  PseudoPeriodic=off  Frequencies=[]  NoiseDistribution=none  NoiseParameters=[]  Unit=1  AffineConversion=off  InputFiltering=off  SimscapeFilterOrder=1  InputFilterTimeConstant=0.001  UdotUserProvided=1
  S-PS2 : nesl_utility/Simulink-PS Converter  PhysicalDomain=network_engine_domain  SubClassName=ps_input  LeftPortType=input  RightPortType=output  PseudoPeriodic=off  Frequencies=[]  NoiseDistribution=none  NoiseParameters=[]  Unit=1  AffineConversion=off  InputFiltering=off  SimscapeFilterOrder=1  InputFilterTimeConstant=0.001  UdotUserProvided=1
  S-PS5 : nesl_utility/Simulink-PS Converter  PhysicalDomain=network_engine_domain  SubClassName=ps_input  LeftPortType=input  RightPortType=output  PseudoPeriodic=off  Frequencies=[]  NoiseDistribution=none  NoiseParameters=[]  Unit=1  AffineConversion=off  InputFiltering=off  SimscapeFilterOrder=1  InputFilterTimeConstant=0.001  UdotUserProvided=1
  Scope : Scope
  Scope1 : Scope
  Simscape Solar Panel : SimscapeComponentBlock  SourceFile=simscape.solarPanel  ComponentPath=simscape.solarPanel  ComponentVariants=simscape.solarPanel  ComponentVariantNames=solarPanel  ClassName=solarPanel  SchemaVersion=1  Rs=1 Ohm  A=2  Iph0=0.050 A  Np=5  Ns=8  Npp=1  efficiency=0.93  i_specify=off  i_priority=None  i=0 A  v_specify=off  v_priority=None  v=0 V
      settings: CopyFcn=simscape.engine.sli.internal.componentblockcallback(gcbh,'COPY')  PreCopyFcn=simscape.engine.sli.internal.componentblockcallback(gcbh,'PRECOPY')  PreDeleteFcn=simscape.engine.sli.internal.componentblockcallback(gcbh,'PREDELETE')
      mask Type: solarPanel
      mask Display:
      | disp('Simscape\n\n\n')
      | disp('\n\n\nsolarPanel');
      | color('red');
      | port_label('LConn', 5,'n');
      | port_label('LConn', 4,'p');
      | port_label('LConn', 3,'diode saturation current');
      | port_label('LConn', 2,'parallel resistance');
      | port_label('LConn', 1,'I');
  + : PMIOPort  Port=1  Side=Left
  - : PMIOPort  Port=2  Side=Left
  wires:
  In1/1 -> If/1, S-PS2/1
  If/1 -> If Action Subsystem/Action
  Rsh/1 -> If Action Subsystem/1(In1)
  Io/1 -> If Action Subsystem/2(In2)
  If/2 -> If Action Subsystem1/Action
  Io1/1 -> If Action Subsystem1/2(In2)
  Rsh1/1 -> If Action Subsystem1/1(In1)
  If Action Subsystem1/1(Out1) -> Merge/2
  If Action Subsystem/1(Out1) -> Merge/1
  Merge/1 -> Scope/1, S-PS1/1
  If/3 -> If Action Subsystem2/Action
  Rsh2/1 -> If Action Subsystem2/1(In1)
  Io2/1 -> If Action Subsystem2/2(In2)
  If Action Subsystem2/1(Out1) -> Merge/3
  If Action Subsystem/2(Out2) -> Merge1/1
  If Action Subsystem1/2(Out2) -> Merge1/2
  If Action Subsystem2/2(Out2) -> Merge1/3
  Merge1/1 -> Scope1/1, S-PS5/1
  connections:
  +/RConn1 -- Simscape Solar Panel/LConn4
  Simscape Solar Panel/LConn5 -- -/RConn1
  S-PS1/RConn1 -- Simscape Solar Panel/LConn2
  Simscape Solar Panel/LConn3 -- S-PS5/RConn1
  S-PS2/RConn1 -- Simscape Solar Panel/LConn1

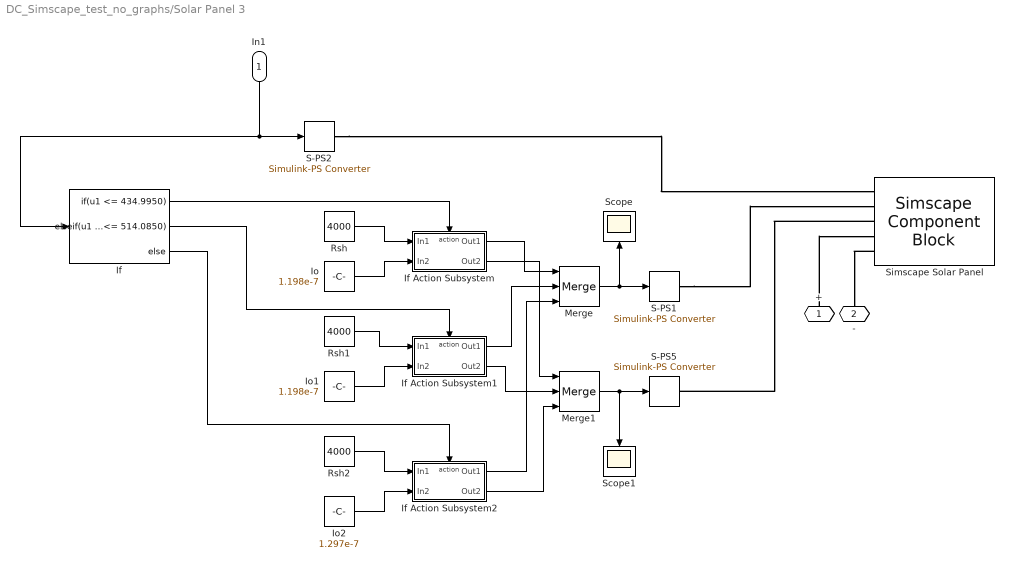
== system DC_Simscape_test_no_graphs/Solar Panel 3 ==
  In1 : Inport
  If : If  IfExpression=u1 <= 434.9950  ElseIfExpressions=u1 <= 514.0850
  If Action Subsystem : Subsystem  TreatAsAtomicUnit=on
  If Action Subsystem1 : Subsystem  TreatAsAtomicUnit=on
  If Action Subsystem2 : Subsystem  TreatAsAtomicUnit=on
  Io : Constant  Value=1.198e-7
  Io1 : Constant  Value=1.198e-7
  Io2 : Constant  Value=1.297e-7
  Merge : Merge  Inputs=3
  Merge1 : Merge  Inputs=3
  Rsh : Constant  Value=4000
  Rsh1 : Constant  Value=4000
  Rsh2 : Constant  Value=4000
  S-PS1 : nesl_utility/Simulink-PS Converter  PhysicalDomain=network_engine_domain  SubClassName=ps_input  LeftPortType=input  RightPortType=output  PseudoPeriodic=off  Frequencies=[]  NoiseDistribution=none  NoiseParameters=[]  Unit=1  AffineConversion=off  InputFiltering=off  SimscapeFilterOrder=1  InputFilterTimeConstant=0.001  UdotUserProvided=1
  S-PS2 : nesl_utility/Simulink-PS Converter  PhysicalDomain=network_engine_domain  SubClassName=ps_input  LeftPortType=input  RightPortType=output  PseudoPeriodic=off  Frequencies=[]  NoiseDistribution=none  NoiseParameters=[]  Unit=1  AffineConversion=off  InputFiltering=off  SimscapeFilterOrder=1  InputFilterTimeConstant=0.001  UdotUserProvided=1
  S-PS5 : nesl_utility/Simulink-PS Converter  PhysicalDomain=network_engine_domain  SubClassName=ps_input  LeftPortType=input  RightPortType=output  PseudoPeriodic=off  Frequencies=[]  NoiseDistribution=none  NoiseParameters=[]  Unit=1  AffineConversion=off  InputFiltering=off  SimscapeFilterOrder=1  InputFilterTimeConstant=0.001  UdotUserProvided=1
  Scope : Scope
  Scope1 : Scope
  Simscape Solar Panel : SimscapeComponentBlock  SourceFile=simscape.solarPanel  ComponentPath=simscape.solarPanel  ComponentVariants=simscape.solarPanel  ComponentVariantNames=solarPanel  ClassName=solarPanel  SchemaVersion=1  Rs=1 Ohm  A=2  Iph0=0.050 A  Np=5  Ns=8  Npp=1  efficiency=0.93  i_specify=off  i_priority=None  i=0 A  v_specify=off  v_priority=None  v=0 V
      settings: CopyFcn=simscape.engine.sli.internal.componentblockcallback(gcbh,'COPY')  PreCopyFcn=simscape.engine.sli.internal.componentblockcallback(gcbh,'PRECOPY')  PreDeleteFcn=simscape.engine.sli.internal.componentblockcallback(gcbh,'PREDELETE')
      mask Type: solarPanel
      mask Display:
      | disp('Simscape\n\n\n')
      | disp('\n\n\nsolarPanel');
      | color('red');
      | port_label('LConn', 5,'n');
      | port_label('LConn', 4,'p');
      | port_label('LConn', 3,'diode saturation current');
      | port_label('LConn', 2,'parallel resistance');
      | port_label('LConn', 1,'I');
  + : PMIOPort  Port=1  Side=Left
  - : PMIOPort  Port=2  Side=Left
  wires:
  In1/1 -> If/1, S-PS2/1
  If/1 -> If Action Subsystem/Action
  Rsh/1 -> If Action Subsystem/1(In1)
  Io/1 -> If Action Subsystem/2(In2)
  If/2 -> If Action Subsystem1/Action
  Io1/1 -> If Action Subsystem1/2(In2)
  Rsh1/1 -> If Action Subsystem1/1(In1)
  If Action Subsystem1/1(Out1) -> Merge/2
  If Action Subsystem/1(Out1) -> Merge/1
  Merge/1 -> Scope/1, S-PS1/1
  If/3 -> If Action Subsystem2/Action
  Rsh2/1 -> If Action Subsystem2/1(In1)
  Io2/1 -> If Action Subsystem2/2(In2)
  If Action Subsystem2/1(Out1) -> Merge/3
  If Action Subsystem/2(Out2) -> Merge1/1
  If Action Subsystem1/2(Out2) -> Merge1/2
  If Action Subsystem2/2(Out2) -> Merge1/3
  Merge1/1 -> Scope1/1, S-PS5/1
  connections:
  +/RConn1 -- Simscape Solar Panel/LConn4
  Simscape Solar Panel/LConn5 -- -/RConn1
  S-PS1/RConn1 -- Simscape Solar Panel/LConn2
  Simscape Solar Panel/LConn3 -- S-PS5/RConn1
  S-PS2/RConn1 -- Simscape Solar Panel/LConn1

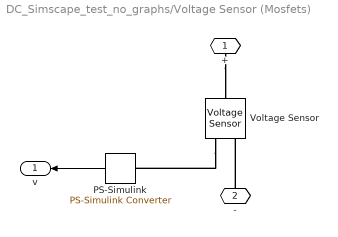
== system DC_Simscape_test_no_graphs/Voltage Sensor (Mosfets) ==
  PS-Simulink : nesl_utility/PS-Simulink Converter  PhysicalDomain=network_engine_domain  SubClassName=ps_output  LeftPortType=input  RightPortType=output  PseudoPeriodic=off  Frequencies=[]  Unit=V  AffineConversion=off
  Voltage Sensor : fl_lib/Electrical/Electrical Sensors/Voltage Sensor
  + : PMIOPort  Port=1  Side=Left
  - : PMIOPort  Port=2  Side=Left
  v : Outport
  wires:
  PS-Simulink/1 -> v/1
  connections:
  -/RConn1 -- Voltage Sensor/RConn2
  +/RConn1 -- Voltage Sensor/LConn1
  Voltage Sensor/RConn1 -- PS-Simulink/LConn1

== system DC_Simscape_test_no_graphs/Voltage Sensor (Resistor BM) ==
  PS-Simulink : nesl_utility/PS-Simulink Converter  PhysicalDomain=network_engine_domain  SubClassName=ps_output  LeftPortType=input  RightPortType=output  PseudoPeriodic=off  Frequencies=[]  Unit=V  AffineConversion=off
  Voltage Sensor : fl_lib/Electrical/Electrical Sensors/Voltage Sensor
  + : PMIOPort  Port=1  Side=Left
  - : PMIOPort  Port=2  Side=Left
  v : Outport
  wires:
  PS-Simulink/1 -> v/1
  connections:
  -/RConn1 -- Voltage Sensor/RConn2
  +/RConn1 -- Voltage Sensor/LConn1
  Voltage Sensor/RConn1 -- PS-Simulink/LConn1

== system DC_Simscape_test_no_graphs/Voltage Sensor Diode Panel 1 ==
  PS-Simulink : nesl_utility/PS-Simulink Converter  PhysicalDomain=network_engine_domain  SubClassName=ps_output  LeftPortType=input  RightPortType=output  PseudoPeriodic=off  Frequencies=[]  Unit=V  AffineConversion=off
  Voltage Sensor : fl_lib/Electrical/Electrical Sensors/Voltage Sensor
  + : PMIOPort  Port=1  Side=Left
  - : PMIOPort  Port=2  Side=Left
  v : Outport
  wires:
  PS-Simulink/1 -> v/1
  connections:
  -/RConn1 -- Voltage Sensor/RConn2
  +/RConn1 -- Voltage Sensor/LConn1
  Voltage Sensor/RConn1 -- PS-Simulink/LConn1

== system DC_Simscape_test_no_graphs/Voltage Sensor Diode Panel 2 ==
  PS-Simulink : nesl_utility/PS-Simulink Converter  PhysicalDomain=network_engine_domain  SubClassName=ps_output  LeftPortType=input  RightPortType=output  PseudoPeriodic=off  Frequencies=[]  Unit=V  AffineConversion=off
  Voltage Sensor : fl_lib/Electrical/Electrical Sensors/Voltage Sensor
  + : PMIOPort  Port=1  Side=Left
  - : PMIOPort  Port=2  Side=Left
  v : Outport
  wires:
  PS-Simulink/1 -> v/1
  connections:
  -/RConn1 -- Voltage Sensor/RConn2
  +/RConn1 -- Voltage Sensor/LConn1
  Voltage Sensor/RConn1 -- PS-Simulink/LConn1

== system DC_Simscape_test_no_graphs/Voltage Sensor Diode Panel 3 ==
  PS-Simulink : nesl_utility/PS-Simulink Converter  PhysicalDomain=network_engine_domain  SubClassName=ps_output  LeftPortType=input  RightPortType=output  PseudoPeriodic=off  Frequencies=[]  Unit=V  AffineConversion=off
  Voltage Sensor : fl_lib/Electrical/Electrical Sensors/Voltage Sensor
  + : PMIOPort  Port=1  Side=Left
  - : PMIOPort  Port=2  Side=Left
  v : Outport
  wires:
  PS-Simulink/1 -> v/1
  connections:
  -/RConn1 -- Voltage Sensor/RConn2
  +/RConn1 -- Voltage Sensor/LConn1
  Voltage Sensor/RConn1 -- PS-Simulink/LConn1

== system DC_Simscape_test_no_graphs/Voltage Sensor Sense Resistor Panel 1  ==
  PS-Simulink : nesl_utility/PS-Simulink Converter  PhysicalDomain=network_engine_domain  SubClassName=ps_output  LeftPortType=input  RightPortType=output  PseudoPeriodic=off  Frequencies=[]  Unit=V  AffineConversion=off
  Voltage Sensor : fl_lib/Electrical/Electrical Sensors/Voltage Sensor
  + : PMIOPort  Port=1  Side=Left
  - : PMIOPort  Port=2  Side=Left
  v : Outport
  wires:
  PS-Simulink/1 -> v/1
  connections:
  -/RConn1 -- Voltage Sensor/RConn2
  +/RConn1 -- Voltage Sensor/LConn1
  Voltage Sensor/RConn1 -- PS-Simulink/LConn1

== system DC_Simscape_test_no_graphs/Voltage Sensor Sense Resistor Panel 2 ==
  PS-Simulink : nesl_utility/PS-Simulink Converter  PhysicalDomain=network_engine_domain  SubClassName=ps_output  LeftPortType=input  RightPortType=output  PseudoPeriodic=off  Frequencies=[]  Unit=V  AffineConversion=off
  Voltage Sensor : fl_lib/Electrical/Electrical Sensors/Voltage Sensor
  + : PMIOPort  Port=1  Side=Left
  - : PMIOPort  Port=2  Side=Left
  v : Outport
  wires:
  PS-Simulink/1 -> v/1
  connections:
  -/RConn1 -- Voltage Sensor/RConn2
  +/RConn1 -- Voltage Sensor/LConn1
  Voltage Sensor/RConn1 -- PS-Simulink/LConn1

== system DC_Simscape_test_no_graphs/Voltage Sensor Sense Resistor Panel 3 ==
  PS-Simulink : nesl_utility/PS-Simulink Converter  PhysicalDomain=network_engine_domain  SubClassName=ps_output  LeftPortType=input  RightPortType=output  PseudoPeriodic=off  Frequencies=[]  Unit=V  AffineConversion=off
  Voltage Sensor : fl_lib/Electrical/Electrical Sensors/Voltage Sensor
  + : PMIOPort  Port=1  Side=Left
  - : PMIOPort  Port=2  Side=Left
  v : Outport
  wires:
  PS-Simulink/1 -> v/1
  connections:
  -/RConn1 -- Voltage Sensor/RConn2
  +/RConn1 -- Voltage Sensor/LConn1
  Voltage Sensor/RConn1 -- PS-Simulink/LConn1

== system DC_Simscape_test_no_graphs/Voltage Sensor Solar Panel 1 ==
  PS-Simulink : nesl_utility/PS-Simulink Converter  PhysicalDomain=network_engine_domain  SubClassName=ps_output  LeftPortType=input  RightPortType=output  PseudoPeriodic=off  Frequencies=[]  Unit=V  AffineConversion=off
  Voltage Sensor : fl_lib/Electrical/Electrical Sensors/Voltage Sensor
  + : PMIOPort  Port=1  Side=Left
  - : PMIOPort  Port=2  Side=Left
  v : Outport
  wires:
  PS-Simulink/1 -> v/1
  connections:
  -/RConn1 -- Voltage Sensor/RConn2
  +/RConn1 -- Voltage Sensor/LConn1
  Voltage Sensor/RConn1 -- PS-Simulink/LConn1

== system DC_Simscape_test_no_graphs/Voltage Sensor Solar Panel 2 ==
  PS-Simulink : nesl_utility/PS-Simulink Converter  PhysicalDomain=network_engine_domain  SubClassName=ps_output  LeftPortType=input  RightPortType=output  PseudoPeriodic=off  Frequencies=[]  Unit=V  AffineConversion=off
  Voltage Sensor : fl_lib/Electrical/Electrical Sensors/Voltage Sensor
  + : PMIOPort  Port=1  Side=Left
  - : PMIOPort  Port=2  Side=Left
  v : Outport
  wires:
  PS-Simulink/1 -> v/1
  connections:
  -/RConn1 -- Voltage Sensor/RConn2
  +/RConn1 -- Voltage Sensor/LConn1
  Voltage Sensor/RConn1 -- PS-Simulink/LConn1

== system DC_Simscape_test_no_graphs/Voltage Sensor Solar Panel 3 ==
  PS-Simulink : nesl_utility/PS-Simulink Converter  PhysicalDomain=network_engine_domain  SubClassName=ps_output  LeftPortType=input  RightPortType=output  PseudoPeriodic=off  Frequencies=[]  Unit=V  AffineConversion=off
  Voltage Sensor : fl_lib/Electrical/Electrical Sensors/Voltage Sensor
  + : PMIOPort  Port=1  Side=Left
  - : PMIOPort  Port=2  Side=Left
  v : Outport
  wires:
  PS-Simulink/1 -> v/1
  connections:
  -/RConn1 -- Voltage Sensor/RConn2
  +/RConn1 -- Voltage Sensor/LConn1
  Voltage Sensor/RConn1 -- PS-Simulink/LConn1

== system DC_Simscape_test_no_graphs/ Battery/ SOC  ==
  PS-Simulink Converter1 : nesl_utility/PS-Simulink Converter  PhysicalDomain=network_engine_domain  SubClassName=ps_output  LeftPortType=input  RightPortType=output  PseudoPeriodic=off  Frequencies=[]  Unit=1  AffineConversion=off
  PS : PMIOPort  Port=1  Side=Left
  tag scope: SOC=global
  wires:
  PS-Simulink Converter1/1 -> [SOC]
  connections:
  PS/RConn1 -- PS-Simulink Converter1/LConn1

== system DC_Simscape_test_no_graphs/ Load/Current Sensor (Load)1 ==
  Current Sensor : fl_lib/Electrical/Electrical Sensors/Current Sensor
  PS-Simulink : nesl_utility/PS-Simulink Converter  PhysicalDomain=network_engine_domain  SubClassName=ps_output  LeftPortType=input  RightPortType=output  PseudoPeriodic=off  Frequencies=[]  Unit=A  AffineConversion=off
  + : PMIOPort  Port=1  Side=Left
  - : PMIOPort  Port=2  Side=Left
  i : Outport
  wires:
  PS-Simulink/1 -> i/1
  connections:
  -/RConn1 -- Current Sensor/RConn2
  +/RConn1 -- Current Sensor/LConn1
  Current Sensor/RConn1 -- PS-Simulink/LConn1

== system DC_Simscape_test_no_graphs/ Load/Current Sensor (Load)2 ==
  Current Sensor : fl_lib/Electrical/Electrical Sensors/Current Sensor
  PS-Simulink : nesl_utility/PS-Simulink Converter  PhysicalDomain=network_engine_domain  SubClassName=ps_output  LeftPortType=input  RightPortType=output  PseudoPeriodic=off  Frequencies=[]  Unit=A  AffineConversion=off
  + : PMIOPort  Port=1  Side=Left
  - : PMIOPort  Port=2  Side=Left
  i : Outport
  wires:
  PS-Simulink/1 -> i/1
  connections:
  -/RConn1 -- Current Sensor/RConn2
  +/RConn1 -- Current Sensor/LConn1
  Current Sensor/RConn1 -- PS-Simulink/LConn1

== system DC_Simscape_test_no_graphs/ Load/Voltage Sensor (Diode)1 ==
  PS-Simulink : nesl_utility/PS-Simulink Converter  PhysicalDomain=network_engine_domain  SubClassName=ps_output  LeftPortType=input  RightPortType=output  PseudoPeriodic=off  Frequencies=[]  Unit=V  AffineConversion=off
  Voltage Sensor : fl_lib/Electrical/Electrical Sensors/Voltage Sensor
  + : PMIOPort  Port=1  Side=Left
  - : PMIOPort  Port=2  Side=Left
  v : Outport
  wires:
  PS-Simulink/1 -> v/1
  connections:
  -/RConn1 -- Voltage Sensor/RConn2
  +/RConn1 -- Voltage Sensor/LConn1
  Voltage Sensor/RConn1 -- PS-Simulink/LConn1

== system DC_Simscape_test_no_graphs/ Load/Voltage Sensor (Diode)4 ==
  PS-Simulink : nesl_utility/PS-Simulink Converter  PhysicalDomain=network_engine_domain  SubClassName=ps_output  LeftPortType=input  RightPortType=output  PseudoPeriodic=off  Frequencies=[]  Unit=V  AffineConversion=off
  Voltage Sensor : fl_lib/Electrical/Electrical Sensors/Voltage Sensor
  + : PMIOPort  Port=1  Side=Left
  - : PMIOPort  Port=2  Side=Left
  v : Outport
  wires:
  PS-Simulink/1 -> v/1
  connections:
  -/RConn1 -- Voltage Sensor/RConn2
  +/RConn1 -- Voltage Sensor/LConn1
  Voltage Sensor/RConn1 -- PS-Simulink/LConn1

== system DC_Simscape_test_no_graphs/Solar Panel 1/If Action Subsystem ==
  In1 : Inport
  In2 : Inport  Port=2
  Action Port : ActionPort  ActionType=then
  Out1 : Outport
  Out2 : Outport  Port=2
  wires:
  In1/1 -> Out1/1
  In2/1 -> Out2/1

== system DC_Simscape_test_no_graphs/Solar Panel 1/If Action Subsystem1 ==
  In1 : Inport
  In2 : Inport  Port=2
  Action Port : ActionPort  ActionType=elseif
  Out1 : Outport
  Out2 : Outport  Port=2
  wires:
  In1/1 -> Out1/1
  In2/1 -> Out2/1

== system DC_Simscape_test_no_graphs/Solar Panel 1/If Action Subsystem2 ==
  In1 : Inport
  In2 : Inport  Port=2
  Action Port : ActionPort  ActionType=else
  Out1 : Outport
  Out2 : Outport  Port=2
  wires:
  In1/1 -> Out1/1
  In2/1 -> Out2/1

== system DC_Simscape_test_no_graphs/Solar Panel 2/If Action Subsystem ==
  In1 : Inport
  In2 : Inport  Port=2
  Action Port : ActionPort  ActionType=then
  Out1 : Outport
  Out2 : Outport  Port=2
  wires:
  In1/1 -> Out1/1
  In2/1 -> Out2/1

== system DC_Simscape_test_no_graphs/Solar Panel 2/If Action Subsystem1 ==
  In1 : Inport
  In2 : Inport  Port=2
  Action Port : ActionPort  ActionType=elseif
  Out1 : Outport
  Out2 : Outport  Port=2
  wires:
  In1/1 -> Out1/1
  In2/1 -> Out2/1

== system DC_Simscape_test_no_graphs/Solar Panel 2/If Action Subsystem2 ==
  In1 : Inport
  In2 : Inport  Port=2
  Action Port : ActionPort  ActionType=else
  Out1 : Outport
  Out2 : Outport  Port=2
  wires:
  In1/1 -> Out1/1
  In2/1 -> Out2/1

== system DC_Simscape_test_no_graphs/Solar Panel 3/If Action Subsystem ==
  In1 : Inport
  In2 : Inport  Port=2
  Action Port : ActionPort  ActionType=then
  Out1 : Outport
  Out2 : Outport  Port=2
  wires:
  In1/1 -> Out1/1
  In2/1 -> Out2/1

== system DC_Simscape_test_no_graphs/Solar Panel 3/If Action Subsystem1 ==
  In1 : Inport
  In2 : Inport  Port=2
  Action Port : ActionPort  ActionType=elseif
  Out1 : Outport
  Out2 : Outport  Port=2
  wires:
  In1/1 -> Out1/1
  In2/1 -> Out2/1

== system DC_Simscape_test_no_graphs/Solar Panel 3/If Action Subsystem2 ==
  In1 : Inport
  In2 : Inport  Port=2
  Action Port : ActionPort  ActionType=else
  Out1 : Outport
  Out2 : Outport  Port=2
  wires:
  In1/1 -> Out1/1
  In2/1 -> Out2/1
